simulink model "AutoExpVideo"  (R2019a)
settings: Solver=FixedStepAuto  StartTime=0.0  StopTime=inf  RelTol=1e-3
undefined symbols (not defined in the file): aeprm_BubblePurgeTime, aeprm_CleanCellTime, aeprm_ExperimentTime, aeprm_GrayValueSetPoint, aeprm_PreparationWaitTime, aeprm_Pump1Speed, aeprm_Pump2Speed, gray
settings Model: EnablePacing=on  Creator=wuyua  LastModifiedBy=wuyua
settings DataIOCC: SaveOutput=off  DSMLogging=off
settings DebuggingCC: ArithmeticOperatorsInVariantConditions=warning

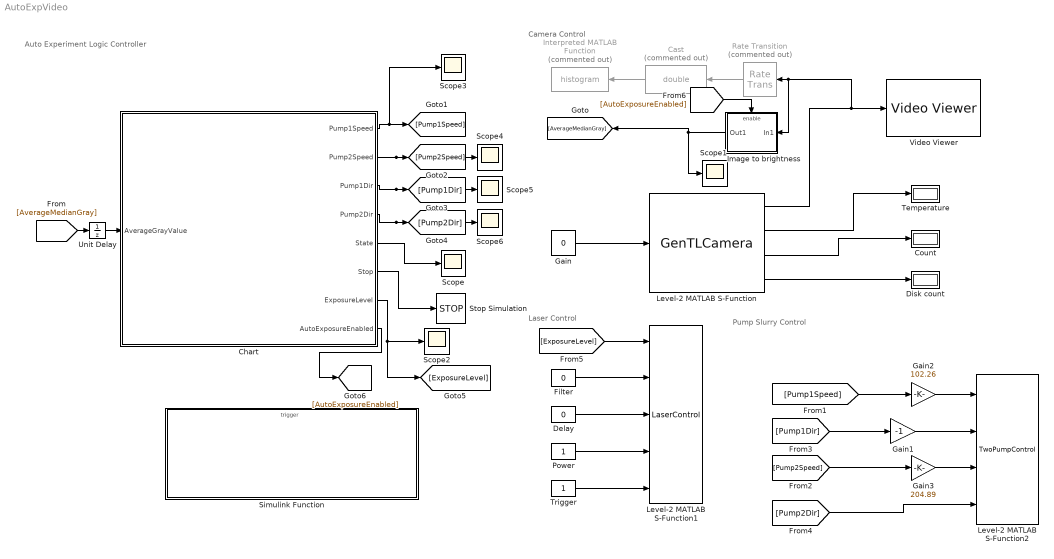
== system AutoExpVideo ==
  note: Auto Experiment Logic Controller
  note: Camera Control
  note: Laser Control
  note: Pump Slurry Control
  Cast : DataTypeConversion  Commented=on  OutDataTypeStr=double
  Chart : Stateflow chart  BlockKeywords=__PRM__SERIALIZED__DATA__:Stateflow Chart,Stateflow Diagram  TreatAsAtomicUnit=on  SystemSampleTime=0.5
  Count : Display
  Delay : Constant  Value=0  OutDataTypeStr=uint32
  Disk count : Display
  Filter : Constant  Value=0  OutDataTypeStr=uint32
  Gain : Constant  Value=0
  Gain1 : Gain  Gain=-1  OutDataTypeStr=int8
  Gain2 : Gain  Gain=102.26
  Gain3 : Gain  Gain=204.89
  Image to brightness : Subsystem
  Interpreted MATLAB Function : MATLABFcn  Commented=on  MATLABFcn=histogram  OutputDimensions=0
  Level-2 MATLAB S-Function : M-S-Function  FunctionName=GenTLCamera
  Level-2 MATLAB S-Function1 : M-S-Function  FunctionName=LaserControl
  Level-2 MATLAB S-Function2 : M-S-Function  FunctionName=TwoPumpControl
  Power : Constant  OutDataTypeStr=uint8
  Rate Transition : RateTransition  Commented=on  OutPortSampleTime=1
  Scope{,1..6} (7 alike) : Scope
  Simulink Function : Subsystem  TreatAsAtomicUnit=on
  Stop Simulation : Stop
  Temperature : Display
  Trigger : Constant  OutDataTypeStr=boolean
  Unit Delay : UnitDelay  SampleTime=-1  HasFrameUpgradeWarning=on
  Video Viewer : VideoViewer  colormapValue=gray(256)  FigPos=[769.8 821.2 766.4 716]
  wires:
  Level-2 MATLAB S-Function/2 -> Temperature/1
  Gain/1 -> Level-2 MATLAB S-Function/1
  Level-2 MATLAB S-Function/1 -> Image to brightness/1(In1), Rate Transition/1, Video Viewer/1
  Filter/1 -> Level-2 MATLAB S-Function1/2
  Delay/1 -> Level-2 MATLAB S-Function1/3
  Power/1 -> Level-2 MATLAB S-Function1/4
  Trigger/1 -> Level-2 MATLAB S-Function1/5
  Gain1/1 -> Level-2 MATLAB S-Function2/2
  [Pump2Dir] -> Level-2 MATLAB S-Function2/4
  Gain3/1 -> Level-2 MATLAB S-Function2/3
  Level-2 MATLAB S-Function/3 -> Count/1
  Level-2 MATLAB S-Function/4 -> Disk count/1
  Rate Transition/1 -> Cast/1
  Cast/1 -> Interpreted MATLAB Function/1
  Image to brightness/1(Out1) -> [AverageMedianGray], Scope1/1
  Gain2/1 -> Level-2 MATLAB S-Function2/1
  [AverageMedianGray] -> Unit Delay/1
  Chart/1(Pump1Speed) -> Scope3/1, [Pump1Speed]
  [Pump1Speed] -> Gain2/1
  Chart/2(Pump2Speed) -> Scope4/1, [Pump2Speed]
  [Pump2Speed] -> Gain3/1
  Chart/3(Pump1Dir) -> Scope5/1, [Pump1Dir]
  Chart/5(State) -> Scope/1
  Chart/6(Stop) -> Stop Simulation/1
  Chart/4(Pump2Dir) -> Scope6/1, [Pump2Dir]
  [Pump1Dir] -> Gain1/1
  Chart/7(ExposureLevel) -> Scope2/1, [ExposureLevel]
  [ExposureLevel] -> Level-2 MATLAB S-Function1/1
  Chart/8(AutoExposureEnabled) -> [AutoExposureEnabled]
  [AutoExposureEnabled] -> Image to brightness/Enable
  Unit Delay/1 -> Chart/1(AverageGrayValue)

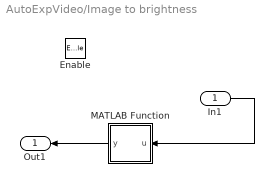
== system AutoExpVideo/Image to brightness ==
  In1 : Inport
  Enable : EnablePort
  MATLAB Function : MATLAB Function  TreatAsAtomicUnit=on  SystemSampleTime=0.5
  Out1 : Outport
  wires:
  In1/1 -> MATLAB Function/1(u)
  MATLAB Function/1(y) -> Out1/1

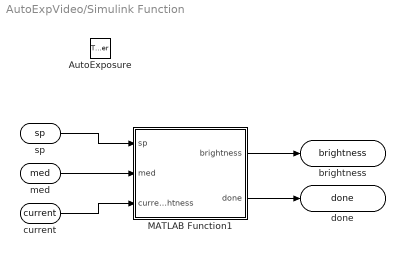
== system AutoExpVideo/Simulink Function ==
  AutoExposure : TriggerPort  TriggerType=function-call  IsSimulinkFunction=on  FunctionName=AutoExposure  VariantControl=(inherit)
  MATLAB Function1 : MATLAB Function  TreatAsAtomicUnit=on
  sp : ArgIn  DisableCoverage=on  ArgumentName=sp
  med : ArgIn  Port=2  ArgumentName=med
  current : ArgIn  Port=3  ArgumentName=current
  brightness : ArgOut  ArgumentName=brightness
  done : ArgOut  Port=2  ArgumentName=done
  wires:
  sp/1 -> MATLAB Function1/1(sp)
  med/1 -> MATLAB Function1/2(med)
  current/1 -> MATLAB Function1/3(currentBrightness)
  MATLAB Function1/1(brightness) -> brightness/1
  MATLAB Function1/2(done) -> done/1

== matlab function AutoExpVideo/Image to brightness/MATLAB Function ==
  data: u input; y output
function y = fcn(u)

y = median(double(u(:)));
% [pixelCounts, grayLevels] = imhist(u,64);
% [~, i] = max(pixelCounts);
% y = grayLevels(i);

== stateflow chart AutoExpVideo/Chart ==
  state INIT
    % Initialize pump speed
    Pump1Speed = 0;
    Pump2Speed = 0;
    % Stop both pump
    Pump1Dir = 0;
    Pump2Dir = 0;
    %Output
    Brightness = 200;
    State = 0;
    Stop = 0;
  state BUBBLE_PURGE
    % Purge bubbles in the flow cell
    Pump1Speed = 2; %2ml/s slurry pump wash
    Pump2Speed = 0.5; % 0.5 ml/s mother liquor wash
    % Stop both pump
    Pump1Dir = 1;
    Pump2Dir = 1;
    State = 1;
  state PREPARATION
    if aeprm_Pump1Speed > 0
    Pump1Speed = aeprm_Pump1Speed;
    else
    Pump1Dir = 0;
    Pump1Speed = 0;
    end
    if aeprm_Pump2Speed > 0
    Pump2Speed = aeprm_Pump2Speed;
    else
    Pump2Dir = 0;
    Pump2Speed = 0;
    end
    State = 2;
  state AUTO_EXPOSURE
    en:
    autoexposure_done = 0;
    AutoExposureEnabled = 1;
    State = 3;
    okFrameCount = 0;
    during:
    [Brightness, autoexposure_done] = AutoExposure(aeprm_GrayValueSetPoint, AverageGrayValue, Brightness);
    ExposureLevel = uint32(Brightness);
    if autoexposure_done
    okFrameCount = okFrameCount + 1;
    else
    okFrameCount = 0;
    end
    exit:
    AutoExposureEnabled = 0;
  state EXPERIMENT_STARTS
    State = 4;
  state FINALIZE
    Pump1Dir = -1;
    Pump2Dir = -1;
  state CLEAN_CELL
    Pump1Dir = -1;
    Pump2Dir = -1;
    Pump1Speed = 0.5; %1ml/s slurry pump wash
    Pump2Speed = 0.5; % 1 ml/s mother liquor wash
    State = 5;
  state STOP_PUMP
    Pump1Dir = 0;
    Pump2Dir = 0;
  state END
    State = 6;
    Stop = 1;
  (default) -> INIT
  INIT -> BUBBLE_PURGE : after(2, sec)
  BUBBLE_PURGE -> PREPARATION : after(aeprm_BubblePurgeTime,sec)
  PREPARATION -> AUTO_EXPOSURE : after(aeprm_PreparationWaitTime, sec)
  AUTO_EXPOSURE -> EXPERIMENT_STARTS : [okFrameCount > 3]
  EXPERIMENT_STARTS -> FINALIZE : after(aeprm_ExperimentTime, sec)
  FINALIZE -> CLEAN_CELL : after(2,sec)
  CLEAN_CELL -> STOP_PUMP : after(aeprm_CleanCellTime,  sec)
  STOP_PUMP -> END : after(1,sec)
  data: aeprm_Pump1Speed parameter; AverageGrayValue input; Pump1Speed output single; Pump2Speed output single; Pump1Dir output int8; Pump2Dir output int8; State output; Stop output; autoexposure_done local; aeprm_Pump2Speed parameter; Brightness local; ExposureLevel output uint32; aeprm_ExperimentTime parameter; aeprm_PreparationWaitTime parameter; aeprm_BubblePurgeTime parameter; aeprm_CleanCellTime parameter; aeprm_GrayValueSetPoint parameter; AutoExposureEnabled output; okFrameCount local

== matlab function AutoExpVideo/Simulink Function/MATLAB Function1 ==
  data: sp input; brightness output; med input; currentBrightness input; done output
function [brightness, done] = fcn(sp, med, currentBrightness)
done = 0;
brightness = currentBrightness;
if med > sp + 10
    brightness = currentBrightness - 20;
elseif med < sp - 10
    brightness = currentBrightness + 20;
else
    done = 1;
end
